simulink model "BatterySim"  (R2021a)
settings: Solver=VariableStepAuto  StartTime=0.0  StopTime=60  FixedStep=60  RelTol=1e-3
settings Model: Creator=jeff  LastModifiedBy=jeff

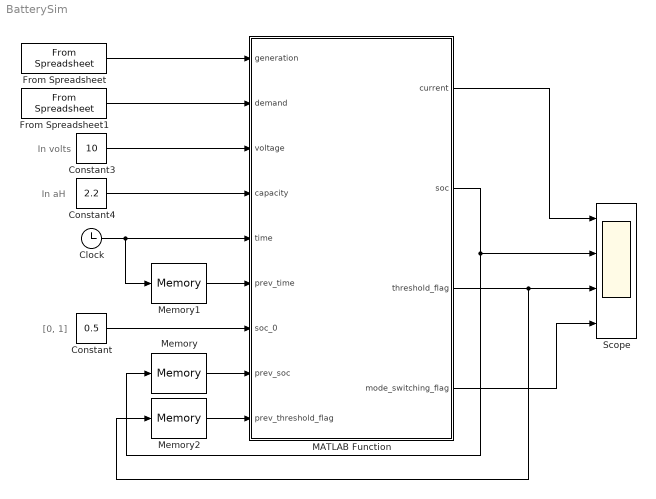
== system BatterySim ==
  note: [0, 1]
  note: In aH
  note: In volts
  Clock : Clock
      settings: Decimation=1000
  Constant : Constant  Value=0.5
  Constant3 : Constant  Value=10
  Constant4 : Constant  Value=2.2
  From Spreadsheet : FromSpreadsheet
  From Spreadsheet1 : FromSpreadsheet
  MATLAB Function : MATLAB Function  TreatAsAtomicUnit=on
  Memory : Memory  InitialCondition=-1
  Memory1 : Memory  InitialCondition=-1
  Memory2 : Memory
  Scope : Scope  NumInputPorts=4
  wires:
  Memory/1 -> MATLAB Function/8(prev_soc)
  MATLAB Function/2(soc) -> Memory/1, Scope/2
  Clock/1 -> Memory1/1, MATLAB Function/5(time)
  Memory1/1 -> MATLAB Function/6(prev_time)
  Constant/1 -> MATLAB Function/7(soc_0)
  Constant3/1 -> MATLAB Function/3(voltage)
  Constant4/1 -> MATLAB Function/4(capacity)
  MATLAB Function/1(current) -> Scope/1
  MATLAB Function/3(threshold_flag) -> Memory2/1, Scope/3
  MATLAB Function/4(mode_switching_flag) -> Scope/4
  Memory2/1 -> MATLAB Function/9(prev_threshold_flag)
  From Spreadsheet/1 -> MATLAB Function/1(generation)
  From Spreadsheet1/1 -> MATLAB Function/2(demand)

== matlab function BatterySim/MATLAB Function ==
  data: generation input; current output; demand input; voltage input; capacity input; time input; prev_time input; soc_0 input; soc output; threshold_flag output; mode_switching_flag output; prev_soc input; prev_threshold_flag input
function [current, soc, threshold_flag, mode_switching_flag] = fcn(generation, demand, voltage, capacity, time, prev_time, soc_0, prev_soc, prev_threshold_flag)
mode_switching_flag = 0;
threshold_flag = 0;

current = (generation-demand)/voltage;

disp(prev_threshold_flag)

if prev_soc == -1 % first iteration
    disp("FIRST");
    soc = soc_0;
else
    if prev_soc < 0.5 && prev_threshold_flag == -1
        disp("LESS THAN 0.5");
        current = generation/voltage;
        threshold_flag = -1;
    elseif prev_soc < 0.3
        disp("CRITICAL")
        current = generation/voltage;
        threshold_flag = -1;
    elseif prev_soc > 0.8 && prev_threshold_flag == 1
        disp("GREATER THAN 0.8");
        current = -1*demand/voltage;
        threshold_flag = 1;
    elseif prev_soc > 0.9
        disp("TOO HIGH")
        current = -1*demand/voltage;
        threshold_flag = 1;
    else
        threshold_flag = 0;
    end
    
    delta_t = time - prev_time;
    current_delta = current*delta_t;
    soc = prev_soc + current_delta/capacity;
    
end
